simulink model "RC_Ckt"  (R2019b)
settings: Solver=VariableStepAuto  StartTime=0.0  StopTime=10.0  RelTol=1e-3
model workspace (MAT data in the model file):
  C = Simulink.Parameter
  C.Value = 1e-05
  C.DataType = 'auto'
  C.Dimensions = [1 1]
  R = Simulink.Parameter
  R.Value = 10
  R.DataType = 'auto'
  R.Dimensions = [1 1]
libraries: fl_lib x2, ee_lib x1
settings Model: Creator=ip  LastModifiedBy=ip

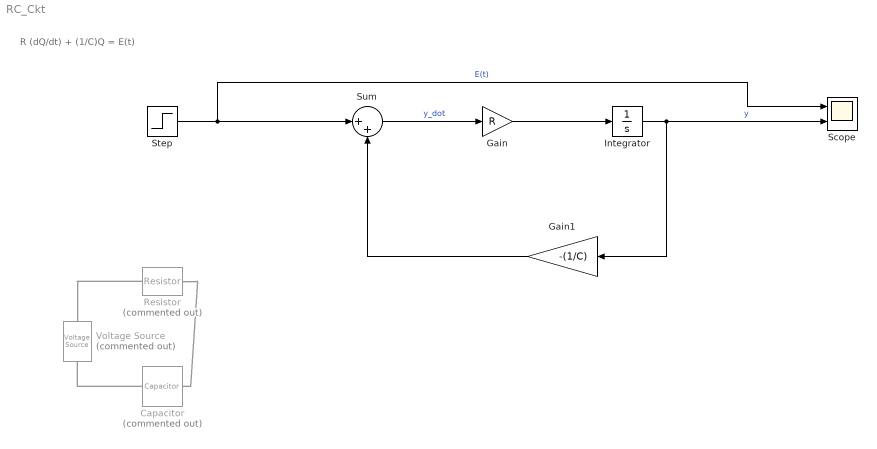
== system RC_Ckt ==
  note: R (dQ/dt) + (1/C)Q = E(t)
  Capacitor : fl_lib/Electrical/Electrical Elements/Capacitor  Commented=on  c=0.00001 F  r=1e-6 Ohm  g=0 1/Ohm  i_specify=off  i_priority=None  i=0 A  i_nominal_specify=off  i_nominal_unit=A  i_nominal_value=1  v_specify=off  v_priority=None  v=0 V  v_nominal_specify=off  v_nominal_unit=V  v_nominal_value=1  vc_specify=off  vc_priority=High  vc=0 V  vc_nominal_specify=off  vc_nominal_unit=V  vc_nominal_value=1
  Gain : Gain  Gain=R
  Gain1 : Gain  Gain=-(1/C)
  Integrator : Integrator
  Resistor : fl_lib/Electrical/Electrical Elements/Resistor  Commented=on  R=10 Ohm  i_specify=off  i_priority=None  i=0 A  i_nominal_specify=off  i_nominal_unit=A  i_nominal_value=1  v_specify=off  v_priority=None  v=0 V  v_nominal_specify=off  v_nominal_unit=V  v_nominal_value=1
  Scope : Scope  NumInputPorts=2
  Step : Step  Time=5  Before=2  SampleTime=0
  Sum : Sum  Inputs=|++
  Voltage Source : ee_lib/Sources/Voltage Source  Commented=on  dc_voltage=0 V  ac_voltage=0 V  ac_shift=0 rad  ac_frequency=60 Hz  noise_mode=0  PSD=0 V^2/Hz  repeatability=1  auto_seed=2816384857  user_seed=0  sample_time=1e-3 s  i_specify=off  i_priority=None  i=0 A  i_nominal_specify=off  i_nominal_unit=A  i_nominal_value=1  v_specify=off  v_priority=None  v=0 V  v_nominal_specify=off  v_nominal_unit=V  v_nominal_value=1
      settings: SourceProductName=Simscape Electrical
  wires:
  Sum/1 -> Gain/1  "y_dot"
  Gain/1 -> Integrator/1
  Integrator/1 -> Scope/2, Gain1/1  "y"
  Gain1/1 -> Sum/2
  Step/1 -> Scope/1, Sum/1  "E(t)"
  connections:
  Resistor/LConn1 -- Voltage Source/LConn1
  Capacitor/LConn1 -- Voltage Source/RConn1
  Resistor/RConn1 -- Capacitor/RConn1
